simulink model "espaco_estados"  (R2018a)
settings: Solver=VariableStepAuto  StartTime=0.0  StopTime=30  RelTol=1e-3
undefined symbols (not defined in the file): A, B, C, D, Fobs, K, Ka, L, offset, Tobs, ts, wt
libraries: arduino_io_lib x5, simulink x1
settings Model: Creator=Mauricio  LastModifiedBy=Mauricio

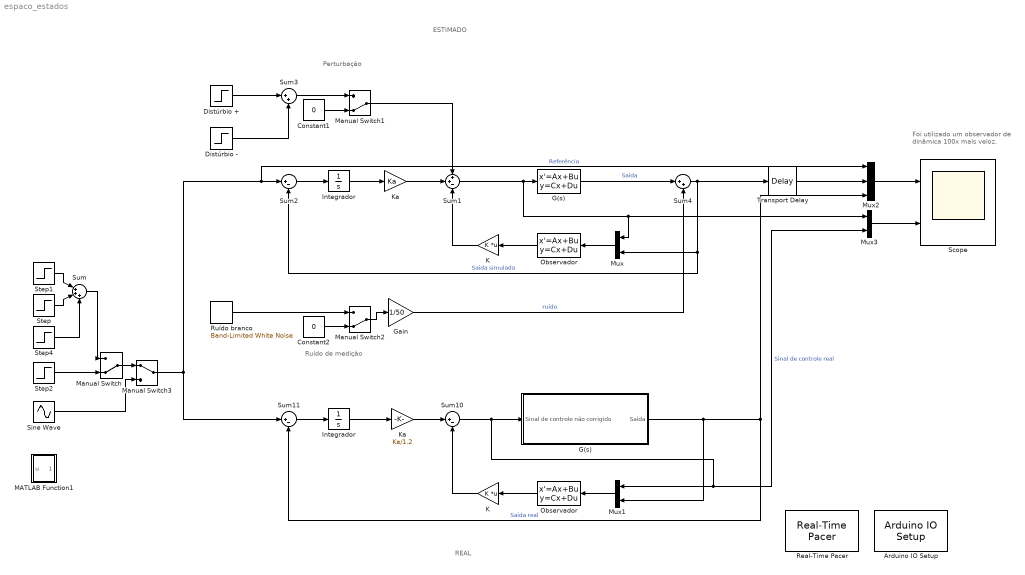
== system espaco_estados ==
  note: Foi utilizado um observador
      | de dinâmica 100x mais veloz.
  note: ESTIMADO
  note: REAL
  note: Ruído de medição
  note: Perturbação
  Arduino IO Setup : arduino_io_lib/Arduino IO Setup  Priority=3  arduinoVar=Temporary arduino variable: Arduino1  workspaceVarName=a  comPort=COM6
  Constant1 : Constant  Value=0
  Constant2 : Constant  Value=0
  Distúrbio + : Step  Time=(ts+wt)*4+offset  After=0.06
  Distúrbio - : Step  Time=(ts+wt)*5+offset  After=-0.06
  G(s) : StateSpace  A=A  B=B  C=C  D=D  InitialCondition=0
  "G(s) " : Subsystem
  Gain : Gain  Gain=1/50
  Integrador : Integrator
  "Integrador " : Integrator
  K : Gain  Gain=K  Multiplication=Matrix(K*u)
  "K " : Gain  Gain=K  Multiplication=Matrix(K*u)
  Ka : Gain  Gain=Ka
  "Ka " : Gain  Gain=Ka/1.2
  MATLAB Function1 : MATLAB Function  TreatAsAtomicUnit=on
  Manual Switch : ManualSwitch  CurrentSetting=0
  Manual Switch1 : ManualSwitch  CurrentSetting=0
  Manual Switch2 : ManualSwitch  CurrentSetting=0
  Manual Switch3 : ManualSwitch
  Mux : Mux  Inputs=2
  Mux1 : Mux  Inputs=2
  Mux2 : Mux  Inputs=3
  Mux3 : Mux  Inputs=2
  Observador : StateSpace  A=Fobs  B=[Tobs*B L]  C=[inv(Tobs)]  D=zeros(size(A,1),2)  InitialCondition=0
  "Observador " : StateSpace  A=Fobs  B=[Tobs*B L]  C=[inv(Tobs)]  D=zeros(size(A,1),2)  InitialCondition=0
  Real-Time Pacer : arduino_io_lib/Real-Time Pacer  simTimePerRealTime=1
  Ruído branco : simulink/Sources/Band-Limited White Noise  Cov=[0.1]  Ts=0.02  seed=[23341]
  Scope : Scope  NumInputPorts=2
  Sine Wave : Sin  Amplitude=6  Frequency=0.5  SampleTime=0.05
  Step : Step  Time=(ts+wt)*1+offset  After=3  SampleTime=0.05
  Step1 : Step  Time=offset  After=3  SampleTime=0.05
  Step2 : Step  Time=0  After=0  SampleTime=0.05
  Step4 : Step  Time=(ts+wt)*2+offset  After=-6  SampleTime=0.05
  Sum : Sum  Inputs=|+++
  Sum1 : Sum  Inputs=++-
  Sum10 : Sum  Inputs=|+-
  Sum11 : Sum  Inputs=|+-
  Sum2 : Sum  Inputs=|+-
  Sum3 : Sum  Inputs=|++
  Sum4 : Sum  Inputs=|++
  Transport Delay : TransportDelay  DelayTime=0.7
  wires:
  Mux3/1 -> Scope/2
  Mux2/1 -> Scope/1
  Sum11/1 -> "Integrador "/1
  Manual Switch3/1 -> Sum11/1, Mux2/1, Sum2/1  "Referência"
  "Integrador "/1 -> "Ka "/1
  Sum4/1 -> Transport Delay/1, Sum2/2, Mux/2  "Saída simulada"
  Ka/1 -> Sum1/2
  Observador/1 -> K/1
  Sum2/1 -> Integrador/1
  K/1 -> Sum1/3
  G(s)/1 -> Sum4/1  "Saída"
  "K "/1 -> Sum10/2
  Mux/1 -> Observador/1
  Integrador/1 -> Ka/1
  Manual Switch1/1 -> Sum1/1
  Distúrbio +/1 -> Sum3/1
  Sum3/1 -> Manual Switch1/1
  Distúrbio -/1 -> Sum3/2
  Constant1/1 -> Manual Switch1/2
  Constant2/1 -> Manual Switch2/2
  Manual Switch2/1 -> Gain/1
  Ruído branco/1 -> Manual Switch2/1
  Gain/1 -> Sum4/2  "ruído"
  "Observador "/1 -> "K "/1
  Mux1/1 -> "Observador "/1
  "G(s) "/1(Saída) -> Mux1/2, Sum11/2, Mux2/3  "Saída real"
  "Ka "/1 -> Sum10/1
  Sum/1 -> Manual Switch/1
  Manual Switch/1 -> Manual Switch3/1
  Step1/1 -> Sum/1
  Step/1 -> Sum/2
  Step2/1 -> Manual Switch/2
  Sine Wave/1 -> Manual Switch3/2
  Step4/1 -> Sum/3
  Sum10/1 -> Mux3/2, Mux1/1, "G(s) "/1(Sinal de controle não corrigido)  "Sinal de controle real"
  Sum1/1 -> G(s)/1, Mux/1, Mux3/1
  Transport Delay/1 -> Mux2/2

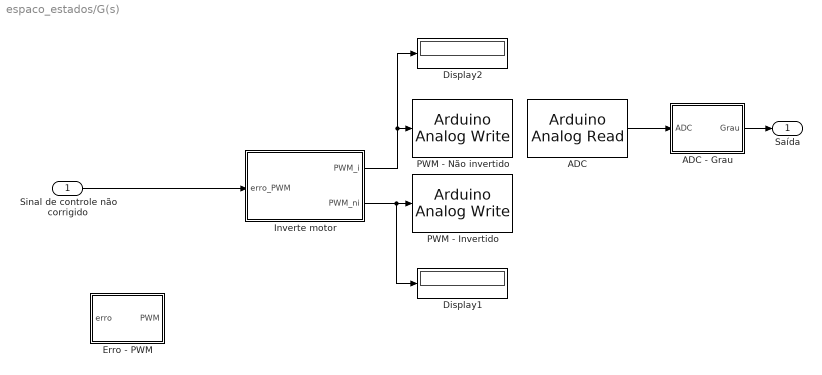
== system espaco_estados/G(s)  ==
  Sinal de controle não corrigido : Inport
  ADC : arduino_io_lib/Arduino Analog Read  arduinoVar=Temporary arduino variable: Arduino1  arduinoPin=2  T=0.01
  ADC - Grau : MATLAB Function  TreatAsAtomicUnit=on
  Display1 : Display
  Display2 : Display
  Erro - PWM : MATLAB Function  TreatAsAtomicUnit=on
  Inverte motor : MATLAB Function  TreatAsAtomicUnit=on
  PWM - Invertido : arduino_io_lib/Arduino Analog Write  arduinoVar=Temporary arduino variable: Arduino1  arduinoPin=6  T=0.05
  PWM - Não invertido : arduino_io_lib/Arduino Analog Write  arduinoVar=Temporary arduino variable: Arduino1  arduinoPin=5  T=0.05
  Saída : Outport
  wires:
  ADC/1 -> ADC - Grau/1(ADC)
  Inverte motor/2(PWM_ni) -> PWM - Invertido/1, Display1/1
  Inverte motor/1(PWM_i) -> Display2/1, PWM - Não invertido/1
  ADC - Grau/1(Grau) -> Saída/1
  Sinal de controle não corrigido/1 -> Inverte motor/1(erro_PWM)

== matlab function espaco_estados/G(s) /Erro - PWM ==
  data: erro input; PWM output
function PWM = fcn(erro)

if(erro < pi/180 && erro >=0)
    PWM = 0;
elseif(erro > -pi/180 && erro < 0)
    PWM = 0;
else
    PWM = 150.7783671396903180968372495108*erro + 57.368421052631578947368421052632;
end

== matlab function espaco_estados/MATLAB Function1 ==
  data: u input; u_ output
function u_ = dead_zone(u)
dz = 45;
if(abs(u)<=dz)
    u_=0;
else
    u_=u;
end

== matlab function espaco_estados/G(s) /ADC - Grau ==
  data: ADC input; Grau output
function Grau = fcn(ADC)
Grau = -0.17413322126497163269594452616096*ADC + 136.2690584156335364572389157386;

== matlab function espaco_estados/G(s) /Inverte motor ==
  data: PWM_i output; PWM_ni output; erro_PWM input
function [PWM_i, PWM_ni] = fcn(erro_PWM)

%REVERSO
if(erro_PWM>0)
    PWM_i = erro_PWM;
    PWM_ni = 0;
%FRENTE
elseif(erro_PWM<0)
    PWM_ni = abs(erro_PWM);
    PWM_i = 0;
%DESLIGADO
else
    PWM_ni = 0;
    PWM_i = 0;
end
